simulink model "SolarEnergy"  (R2020a)
settings: Solver=FixedStepDiscrete  StartTime=0.0  StopTime=20000.0  FixedStep=1  RelTol=1e-3  EnableMultiTasking=on
settings Model: Creator=mbruchanski  LastModifiedBy=ningwersen
settings DataIOCC: LimitDataPoints=on  SaveFormat=Array  InspectSignalLogs=on  ReturnWorkspaceOutputs=off
settings OptimizationCC: LifeSpan=inf
settings DebuggingCC: UnderspecifiedInitializationDetection=Classic  MergeDetectMultiDrivingBlocksExec=none  SolverPrmCheckMsg=warning  MultiTaskDSMMsg=warning  MultiTaskCondExecSysMsg=none  StateNameClashWarn=warning  SFUnexpectedBacktrackingDiag=warning  SFNoUnconditionalDefaultTransitionDiag=warning  SFExecutionAtInitializationDiag=none  ArithmeticOperatorsInVariantConditions=warning
settings HardwareCC: ProdBitPerPointer=32  ProdBitPerSizeT=32  ProdBitPerPtrDiffT=32  ProdLargestAtomicFloat=None  ProdIntDivRoundTo=Undefined  ProdEndianess=Unspecified  ProdWordSize=32  ProdHWDeviceType=32-bit Generic
settings ModelReferenceCC: PropagateSignalLabelsOutOfModel=off
settings SFSimCC: SimUseLocalCustomCode=off  CustomCodeUndefinedFunction=UseInterfaceOnly
settings RTWCC: RTWUseLocalCustomCode=off
settings CodeAppCC: StateflowObjectComments=on
settings GRTTargetCC: TargetLangStandard=C89/C90 (ANSI)
settings ConfigComp: CovMetricSettings=dw  CovHtmlReporting=on  CovSaveCumulativeToWorkspaceVar=on  CovSaveSingleToWorkspaceVar=on  CovExternalEMLEnable=off

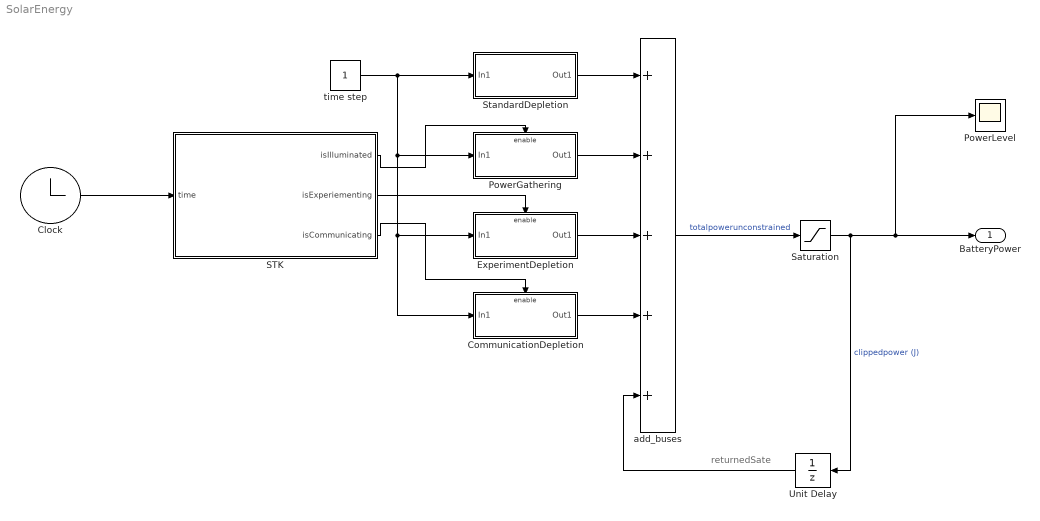
== system SolarEnergy ==
  note: returnedSate
  Clock : Clock
  CommunicationDepletion : Subsystem  TreatAsAtomicUnit=on
  ExperimentDepletion : Subsystem  TreatAsAtomicUnit=on
  PowerGathering : Subsystem  TreatAsAtomicUnit=on
  PowerLevel : Scope
  STK : Subsystem
      mask Display: image(imread('RAX2.jpg'))
  Saturation : Saturate  UpperLimit=96000  LowerLimit=0
  StandardDepletion : Subsystem  TreatAsAtomicUnit=on
  Unit Delay : UnitDelay  InitialCondition=90000  SampleTime=-1  HasFrameUpgradeWarning=on
  add_buses : Sum  Inputs=+++++
  time step : Constant  SampleTime=-1
  BatteryPower : Outport
  wires:
  add_buses/1 -> Saturation/1  "totalpowerunconstrained"
  ExperimentDepletion/1(Out1) -> add_buses/3
  CommunicationDepletion/1(Out1) -> add_buses/4
  Saturation/1 -> Unit Delay/1, PowerLevel/1, BatteryPower/1  "clippedpower (J)"
  Clock/1 -> STK/1(time)
  STK/1(isIlluminated) -> PowerGathering/Enable
  STK/2(isExperiementing) -> ExperimentDepletion/Enable
  STK/3(isCommunicating) -> CommunicationDepletion/Enable
  PowerGathering/1(Out1) -> add_buses/2
  time step/1 -> ExperimentDepletion/1(In1), CommunicationDepletion/1(In1), PowerGathering/1(In1), StandardDepletion/1(In1)
  Unit Delay/1 -> add_buses/5
  StandardDepletion/1(Out1) -> add_buses/1

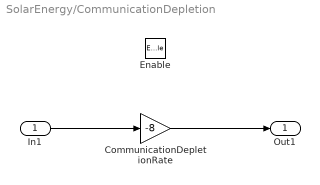
== system SolarEnergy/CommunicationDepletion ==
  In1 : Inport
  Enable : EnablePort
  CommunicationDepletionRate : Gain  Gain=-8
  Out1 : Outport  OutputWhenDisabled=reset  InitialOutput=0
  wires:
  In1/1 -> CommunicationDepletionRate/1
  CommunicationDepletionRate/1 -> Out1/1

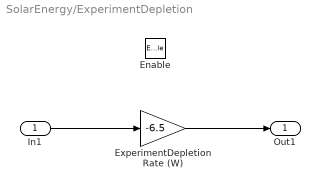
== system SolarEnergy/ExperimentDepletion ==
  In1 : Inport
  Enable : EnablePort
  ExperimentDepletionRate (W) : Gain  Gain=-6.5
  Out1 : Outport  OutputWhenDisabled=reset  InitialOutput=0
  wires:
  In1/1 -> ExperimentDepletionRate (W)/1
  ExperimentDepletionRate (W)/1 -> Out1/1

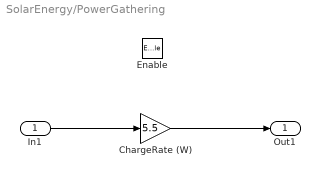
== system SolarEnergy/PowerGathering ==
  In1 : Inport
  Enable : EnablePort  StatesWhenEnabling=reset
  ChargeRate (W) : Gain  Gain=5.5
  Out1 : Outport  OutputWhenDisabled=reset  InitialOutput=0
  wires:
  In1/1 -> ChargeRate (W)/1
  ChargeRate (W)/1 -> Out1/1

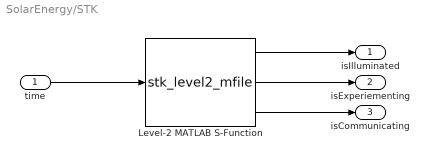
== system SolarEnergy/STK ==
  time : Inport
  Level-2 MATLAB S-Function : M-S-Function  InitFcn=|  FunctionName=stk_level2_mfile
      | %create a new instance of STK12                                                                                                                   
      | uiapp = actxserver('STK12.application');                                                                                                          
      | root = uiapp.Personality2;                                                                                                                        
      | uiapp.visible = 1;             
      |                                                                                                                    
      | %create a new scenario and specify the time                                                                                                       
      | root.NewScenario('SimulinkRun');   
      | scenario = root.CurrentScenario;                                                                                                               
      | root.UnitPreferences.Item('DateFormat').SetCurrentUnit('UTCG');                                                                                   
      | scenario.SetTimePeriod('1 Jul 2013 12:00:00.000', '2 Jul 2013 12:00:00.000');                                                         
      | scenario.Epoch = '1 Jul 2013 12:00:00.000';        
      | root.Rewind();
      |                                                                                    
      | %create a new satellite and propagate                                                                                                             
      | satellite = root.CurrentScenario.Children.New('eSatellite', 'ScienceSat');                                                                           
      | satellite.Propagator.InitialState.Representation.AssignClassical('eCoordinateSystemJ2000', 7045.635754, 0.000859, 98.093, 255.746, 213.045, 251.982);
      | satellite.Propagator.EphemerisInterval.SetStartAndStopTimes(scenario.StartTime, scenario.StopTime);                                                                                           
      | satellite.Propagator.Propagate();
      |                                                                                                                       
      | %create a new facility                                                                                                                            
      | facility = root.CurrentScenario.Children.New('eFacility', 'GroundStation');                                                                         
      | facility.Position.AssignPlanetodetic(30.4794, -86.5234, 0);   
      |                                                                                       
      | %add a sensor to the facility and target it at the satellite                                                                                      
      | pointingSensor = facility.Children.New('eSensor', 'Targeted');                                                                                      
      | pointingSensor.Pattern.ConeAngle = 3.0;                                                                                                           
      | pointingSensor.SetPointingType('eSnPtTargeted');                                                                                                  
      | pointingSensor.Pointing.Targets.AddObject(satellite);
      |                                                                                             
      | %add a reciever to the ground station                                                                                                             
      | receiver = pointingSensor.Children.New('eReceiver', 'DownlinkRx');                                                                                      
      | receiver.SetModel('Complex Receiver Model');
      | receiverAntenna = receiver.Model.AntennaControl;
      | receiverAntenna.SetEmbeddedModel('Parabolic');
      | receiverAntenna.EmbeddedModel.Diameter = 3;  % m
      |                                                                                                                                             
      | %add a transmitter to the satellite                                                                                                               
      | transmitter = satellite.Children.New('eTransmitter', 'DownlinkTx');
      | transmitter.SetModel('Complex Transmitter Model');
      | transmitterAntenna = transmitter.Model.AntennaControl;
      | transmitterAntenna.SetEmbeddedModel('Parabolic');
      | transmitterAntenna.EmbeddedModel.Diameter = 0.25;  % m
      | 
      | transmitter.Model.Power = 150;  % dbW
      | transmitter.Model.Frequency = 4.04;  % GHz
      |                                                                                                                                        
      | %Constrain the receiver for max BER 1e-8                                                                                                          
      | berConstraint = receiver.AccessConstraints.AddConstraint('eCstrBitErrorRate');                                                                                    
      | berConstraint.EnableMax = 1;                                                                                                                                
      | berConstraint.Max = 0.00000001;   
      | 
      | % create the Sun                                                                                                                                  
      | sun = root.CurrentScenario.Children.New('ePlanet', 'Sun');        
      | 
      | % add a science sensor on the satellite, define as rectangular 5x5                                                                                
      | scienceSensor = satellite.Children.New('eSensor', 'scienceSensor');                                                                                      
      | scienceSensor.SetPatternType('eSnRectangular');                                                                                                       
      | scienceSensor.Pattern.HorizontalHalfAngle = 5.0;                                                                                                      
      | scienceSensor.Pattern.VerticalHalfAngle = 5.0;      
      | 
      | % create an area target for greenland                                                                                                             
      | result = root.ExecuteCommand('GetDirectory / STKHome');                                                                                           
      | installDirectory = result.Item(0);                                                                                                                      
      | root.ExecuteCommand(['GIS * Import "' installDirectory '\Data\Shapefiles\Countries\Greenland\Greenland.shp" AreaTarget']);                              
      | 
      | %need to remove all those extra area targets                                                                                                      
      | root.ExecuteCommand('UnloadMulti / */AreaTarget/Greenland_*');                                                                                    
      | greenland = root.CurrentScenario.Children.Item('Greenland'); 
      | 
      | %set an elevation constraint on the area target, otherwise the one point                                                                          
      | %access will not work correctly for the sensor.                                                                                                   
      | elevationConstraint = greenland.AccessConstraints.AddConstraint('eCstrElevationAngle');                                                                     
      | elevationConstraint.Angle = 90.0;         
      | 
      | % create an access object from the science sensor to the area target                                                                              
      | greenlandAccess = scienceSensor.CreateOnePointAccess(greenland.Path);  
      | 
      | % create an access object from the satellite to the sun                                                                                           
      | sunAccess = satellite.CreateOnePointAccess(sun.Path); 
      | 
      | % create an access object from the rx to the tx                                                                                                   
      | communicationsAccess = receiver.CreateOnePointAccess(transmitter.Path);      
      | 
      | % set STK to expect times in epoch seconds                                                                                                        
      | root.UnitPreferences.Item('DateFormat').SetCurrentUnit('EpSec');                                                                                  
      | stkParameters = cell(5,1);                                                                                                                      
      | stkParameters{1} = uiapp;                                                                                                                         
      | stkParameters{2} = root;                                                                                                                          
      | stkParameters{3} = sunAccess;                                                                                                                     
      | stkParameters{4} = greenlandAccess;                                                                                                                      
      | stkParameters{5} = communicationsAccess;  
      | 
      | %assign the structure we'll use later to the UserData                                                                                             
      | set_param(gcb,'UserData', stkParameters);
  isIlluminated : Outport
  isExperiementing : Outport  Port=2
  isCommunicating : Outport  Port=3
  wires:
  time/1 -> Level-2 MATLAB S-Function/1
  Level-2 MATLAB S-Function/1 -> isIlluminated/1
  Level-2 MATLAB S-Function/2 -> isExperiementing/1
  Level-2 MATLAB S-Function/3 -> isCommunicating/1

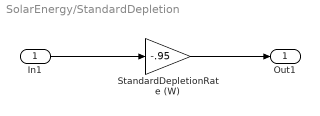
== system SolarEnergy/StandardDepletion ==
  In1 : Inport
  StandardDepletionRate (W) : Gain  Gain=-.95
  Out1 : Outport
  wires:
  In1/1 -> StandardDepletionRate (W)/1
  StandardDepletionRate (W)/1 -> Out1/1
